simulink model "Senorless"  (R2023a)
settings: Solver=FixedStepDiscrete  StartTime=0.0  StopTime=2  FixedStep=1/FOC_FRQ  RelTol=1e-3
values from neighbouring files (symbols this model uses):
  ADC_REF = 3.6    [Senorless.sldd]
  ADC_SAMPLE_MAX = 32767.0    [Senorless.sldd]
  AMP_GAIN = 32.0    [Senorless.sldd]
  CURR_INPUT = 3276.0    [Senorless.sldd]
  CURR_KI = 380.0    [Senorless.sldd]
  CURR_KP = 0.04    [Senorless.sldd]
  CURR_LIMIT = 1.1    [Senorless.sldd]
  CURR_OVER = 34.0    [Senorless.sldd]
  CURR_POINT_GAIN = 7.0    [Senorless.sldd]
  CURR_STEP = 32760.0    [Senorless.sldd]
  CURR_UNDER = 0.03    [Senorless.sldd]
  CURR_WIDTH = 250.0    [Senorless.sldd]
  FOC_FRQ = 36000.0    [Senorless.sldd]
  GAMMA = 32767.0    [Senorless.sldd]
  HFI_ID = 2.125    [Senorless.sldd]
  IMAX = 34.0    [Senorless.sldd]
  LPF_FRQ = 300.0    [Senorless.sldd]
  MOTOR_DAMPER = 8.3E-7    [Senorless.sldd]
  MOTOR_FLUX = 0.0012713112    [Senorless.sldd]
  MOTOR_INERTIA = 1.02E-6    [Senorless.sldd]
  MOTOR_LS = 1.8E-5    [Senorless.sldd]
  MOTOR_PN = 7.0    [Senorless.sldd]
  MOTOR_RS = 0.065    [Senorless.sldd]
  NS_COMP_UD = 0.531    [Senorless.sldd]
  PLL_LIMIT = 0.95    [Senorless.sldd]
  PLL_WIDTH = 500.0    [Senorless.sldd]
  PWM_FRQ = 96000000.0    [Senorless.sldd]
  RS_HUNT = 0.002    [Senorless.sldd]
  SMOK_FRQ = 1200.0    [Senorless.sldd]
  SPD_LIMIT = 0.8    [Senorless.sldd]
  SPD_LPF_LEVEL = 15.0    [Senorless.sldd]
  SPD_MAX = 8100.0    [Senorless.sldd]
  SPD_MIN = -8100.0    [Senorless.sldd]
  SPD_REDUCE = 380.0    [Senorless.sldd]
  SPD_STEP = 3.0    [Senorless.sldd]
  SPD_WIDTH = 10.0    [Senorless.sldd]
  TS_POINT_GAIN = 10.0    [Senorless.sldd]
  UDC = 17.0    [Senorless.sldd]
  UDC_GAIN = 21.0    [Senorless.sldd]
  UDC_POINT_GAIN = 10.0    [Senorless.sldd]
undefined symbols (not defined in the file or in its folder): curr_q_ki, curr_q_kp, DiscIntNeverNeededParam, magnitude, PLL_LPF_LEVEL, Udc
libraries: simulink x20, slpidlib x5, mcbcontrolslib x4, mcbplantlib x1, autolibpmsminterior x1, autolibpmsmexterior x1, spspowerguiLib x1
(part 3 of 7)

== system Senorless/FOC_PointModel/标志位 ==
  NS_Flag : Inport  PortDimensions=1
  Obs_Theta : Inport  Port=2
  Action Port : ActionPort  InitializeStates=reset  ActionPortLabel=case [ 3 ]:
  Constant1 : Constant  Value=0  OutDataTypeStr=int32
  Constant4 : Constant  Value=0  OutDataTypeStr=int16
  Constant8 : Constant  Value=0  OutDataTypeStr=int16
  Data Store Write : DataStoreWrite  DataStoreName=NS_Flag  IndexOptions=Index vector (dialog)  Indices=1  OutputSizes=1
  Data Type Conversion1 : DataTypeConversion  Commented=on  OutDataTypeStr=int32  SaturateOnIntegerOverflow=off
  Data Type Conversion2 : DataTypeConversion  Commented=on  OutDataTypeStr=int32  SaturateOnIntegerOverflow=off
  Display : Display
  Shift Arithmetic : ArithShift  Commented=on  BitShiftNumber=-16
  Sign : Signum
  积分器 : Subsystem  Commented=on
      settings: MinAlgLoopOccurrences=on
  Theta : Outport
  Iq : Outport  Port=2
  Id : Outport  Port=3
  wires:
  Data Type Conversion1/1 -> 积分器/2(Xo)
  Data Type Conversion2/1 -> Shift Arithmetic/1
  Shift Arithmetic/1 -> 积分器/1(input)
  Constant8/1 -> Iq/1
  Constant4/1 -> Id/1
  Obs_Theta/1 -> Theta/1
  NS_Flag/1 -> Sign/1
  Sign/1 -> Display/1, Data Store Write/1

== system Senorless/FOC_PointModel/电压限转速 ==
  note: 通过实时检测母线电压，调整最大转速
  Udc_Ref : Inport
  SPD_Ref : Inport  Port=2
  Constant1 : Constant  Value=SPD_REDUCE  OutDataTypeStr=int32
  Constant2 : Constant  Value=2  OutDataTypeStr=int16
  Constant3 : Constant  Value=0  OutDataTypeStr=int16
  Constant6 : Constant  Value=SPD_MAX  OutDataTypeStr=int32
  Constant7 : Constant  Value=SPD_MIN  OutDataTypeStr=int32
  Data Store Read1 : DataStoreRead  DataStoreName=Uout_Max  IndexOptions=Index vector (dialog)  Indices=1  OutputSizes=1
  Data Store Read2 : DataStoreRead  DataStoreName=Uout_Max  IndexOptions=Index vector (dialog)  Indices=1  OutputSizes=1
  Data Store Read3 : DataStoreRead  DataStoreName=Uout_Max  IndexOptions=Index vector (dialog)  Indices=1  OutputSizes=1
  Product : Product  OutDataTypeStr=int32  RndMeth=Zero
  Product4 : Product  OutDataTypeStr=int32
  Saturation Dynamic1 : simulink/Discontinuities/Saturation Dynamic  OutMin=[]  OutMax=[]  OutDataTypeStr=Inherit: Same as second input  OutDataType=fixdt(1, 16)  OutScaling=2^-10  RndMeth=Zero  DoSatur=off
  Saturation Dynamic2 : simulink/Discontinuities/Saturation Dynamic  OutMin=[]  OutMax=[]  OutDataTypeStr=Inherit: Same as second input  OutDataType=fixdt(1, 16)  OutScaling=2^-10  RndMeth=Zero  DoSatur=off
  Shift Arithmetic : ArithShift  BitShiftNumber=15
  Sum : Sum  Inputs=-+  OutDataTypeStr=int16  RndMeth=Zero
  Sum1 : Sum  Inputs=-+  OutDataTypeStr=int16  RndMeth=Zero
  Sum2 : Sum  Inputs=+-  RndMeth=Zero
  out : Outport
  wires:
  Product4/1 -> Shift Arithmetic/1
  Sum/1 -> Saturation Dynamic1/2
  Shift Arithmetic/1 -> Sum/1
  SPD_Ref/1 -> Saturation Dynamic2/2
  Udc_Ref/1 -> Product4/2
  Sum2/1 -> Saturation Dynamic2/1
  Saturation Dynamic2/1 -> out/1
  Constant7/1 -> Saturation Dynamic2/3
  Constant1/1 -> Product/1
  Saturation Dynamic1/1 -> Product/2
  Constant6/1 -> Sum2/1
  Product/1 -> Sum2/2
  Data Store Read3/1 -> Product4/1
  Sum1/1 -> Sum/2
  Constant2/1 -> Sum1/1
  Data Store Read1/1 -> Sum1/2
  Constant3/1 -> Saturation Dynamic1/3
  Data Store Read2/1 -> Saturation Dynamic1/1

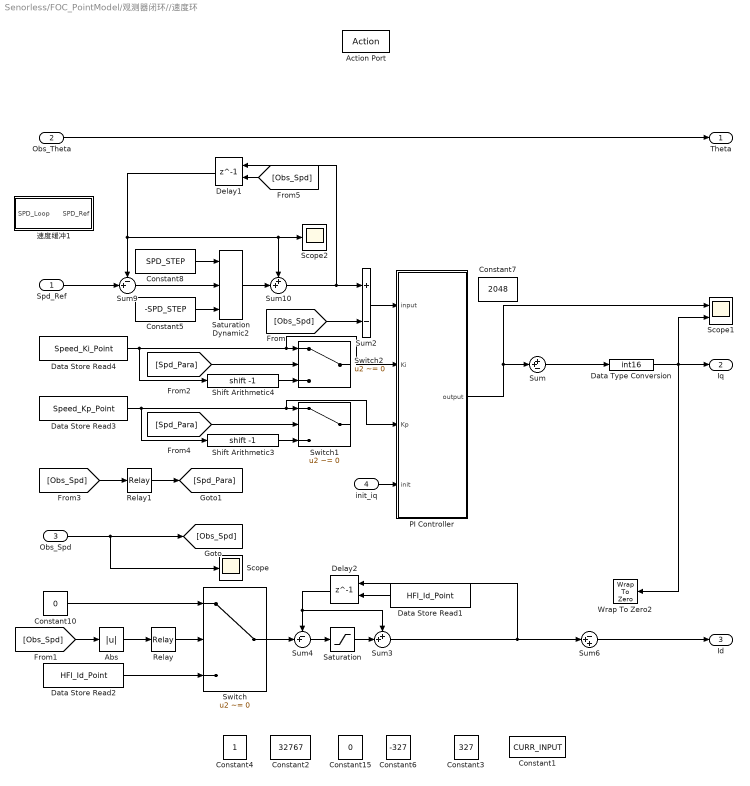
== system Senorless/FOC_PointModel/观测器闭环//速度环 ==
  Spd_Ref : Inport
  Obs_Theta : Inport  Port=2
  Obs_Spd : Inport  Port=3
  init_iq : Inport  Port=4
  Action Port : ActionPort  InitializeStates=reset  ActionPortLabel=case [ 4 ]:
  Abs : Abs  SaturateOnIntegerOverflow=off
  Constant1 : Constant  Value=CURR_INPUT  OutDataTypeStr=int16
  Constant10 : Constant  Value=0  OutDataTypeStr=int16
  Constant15 : Constant  Value=0  OutDataTypeStr=int16
  Constant2 : Constant  Value=32767  OutDataTypeStr=int16
  Constant3 : Constant  Value=327  OutDataTypeStr=int16
  Constant4 : Constant  OutDataTypeStr=int16
  Constant5 : Constant  Value=-SPD_STEP  OutDataTypeStr=int32
  Constant6 : Constant  Value=-327  OutDataTypeStr=int16
  Constant7 : Constant  Value=2048  OutDataTypeStr=int16
  Constant8 : Constant  Value=SPD_STEP  OutDataTypeStr=int32
  Data Store Read1 : DataStoreRead  DataStoreName=HFI_Id_Point  IndexOptions=Index vector (dialog)  Indices=1  OutputSizes=1
  Data Store Read2 : DataStoreRead  DataStoreName=HFI_Id_Point  IndexOptions=Index vector (dialog)  Indices=1  OutputSizes=1
  Data Store Read3 : DataStoreRead  DataStoreName=Speed_Kp_Point  IndexOptions=Index vector (dialog)  Indices=1  OutputSizes=1
  Data Store Read4 : DataStoreRead  DataStoreName=Speed_Ki_Point  IndexOptions=Index vector (dialog)  Indices=1  OutputSizes=1
  Data Type Conversion : DataTypeConversion  OutDataTypeStr=int16  SaturateOnIntegerOverflow=off
  Delay1 : Delay  DelayLength=1  InitialConditionSource=Input port
      settings: InputPortMap=u0,p4
  Delay2 : Delay  DelayLength=1  InitialConditionSource=Input port
      settings: InputPortMap=u0,p4
  PI Controller : Subsystem
      settings: MinAlgLoopOccurrences=on
  Relay : Relay  OnSwitchValue=1700  OffSwitchValue=1300  OnOutputValue=boolean(1)  OffOutputValue=boolean(0)  OutDataTypeStr=boolean
  Relay1 : Relay  OnSwitchValue=150  OffSwitchValue=100  OnOutputValue=boolean(1)  OffOutputValue=boolean(0)  OutDataTypeStr=boolean
  Saturation : Saturate  UpperLimit=16384  LowerLimit=-1
  Saturation Dynamic2 : simulink/Discontinuities/Saturation Dynamic  OutMin=[]  OutMax=[]  OutDataTypeStr=Inherit: Same as second input  OutDataType=fixdt(1, 16)  OutScaling=2^-10  RndMeth=Zero  DoSatur=off
  Scope : Scope
  Scope1 : Scope  NumInputPorts=2
  Scope2 : Scope
  Shift Arithmetic3 : ArithShift  BitShiftNumber=-1
  Shift Arithmetic4 : ArithShift  BitShiftNumber=-1
  Sum : Sum  Inputs=++-  RndMeth=Zero
  Sum10 : Sum  Inputs=++|  OutDataTypeStr=int32  RndMeth=Zero
  Sum2 : Sum  Inputs=+-  AccumDataTypeStr=int32  OutDataTypeStr=int16  RndMeth=Zero
  Sum3 : Sum  Inputs=++|  OutDataTypeStr=int16  RndMeth=Zero
  Sum4 : Sum  Inputs=-+|  OutDataTypeStr=int16  RndMeth=Zero
  Sum6 : Sum  Inputs=-++  OutDataTypeStr=int16  RndMeth=Zero
  Sum9 : Sum  Inputs=-+|  OutDataTypeStr=int32  RndMeth=Zero
  Switch : Switch  Criteria=u2 ~= 0  Threshold=1500  OutDataTypeStr=int16  RndMeth=Zero  SaturateOnIntegerOverflow=off  InputSameDT=off
  Switch1 : Switch  Criteria=u2 ~= 0  Threshold=100  SaturateOnIntegerOverflow=off  InputSameDT=off
  Switch2 : Switch  Criteria=u2 ~= 0  Threshold=100  SaturateOnIntegerOverflow=off  InputSameDT=off
  Wrap To Zero2 : simulink/Discontinuities/Wrap To Zero  Threshold=int16(0)
  速度缓冲1 : Stateflow chart  TreatAsAtomicUnit=on
  Theta : Outport  InitialOutput=uint16(0)
  Iq : Outport  Port=2  InitialOutput=int16(0)
  Id : Outport  Port=3  InitialOutput=int16(0)
  wires:
  Obs_Theta/1 -> Theta/1
  Sum2/1 -> PI Controller/1(input)
  Saturation Dynamic2/1 -> Sum10/2
  Delay1/1 -> Sum10/1, Scope2/1, Sum9/1
  Sum9/1 -> Saturation Dynamic2/2
  Constant8/1 -> Saturation Dynamic2/1
  Constant5/1 -> Saturation Dynamic2/3
  [Obs_Spd] -> Abs/1
  Relay/1 -> Switch/2
  Shift Arithmetic4/1 -> Switch2/3
  Shift Arithmetic3/1 -> Switch1/3
  Data Type Conversion/1 -> Wrap To Zero2/1, Scope1/2, Iq/1
  Sum/1 -> Data Type Conversion/1
  PI Controller/1(output) -> Scope1/1, Sum/2
  Sum3/1 -> Sum6/2, Delay2/1
  Sum4/1 -> Saturation/1
  Saturation/1 -> Sum3/2
  Delay2/1 -> Sum3/1, Sum4/1
  [Obs_Spd] -> Sum2/2
  Switch/1 -> Sum4/2
  [Obs_Spd] -> Relay1/1
  [Spd_Para] -> Switch2/2
  [Spd_Para] -> Switch1/2
  Relay1/1 -> [Spd_Para]
  Constant10/1 -> Switch/1
  Data Store Read4/1 -> Shift Arithmetic4/1, PI Controller/2(Ki), Switch2/1
  Data Store Read3/1 -> PI Controller/3(Kp), Switch1/1, Shift Arithmetic3/1
  Data Store Read2/1 -> Switch/3
  Data Store Read1/1 -> Delay2/2
  Spd_Ref/1 -> Sum9/2
  Sum10/1 -> Delay1/1, Sum2/1
  [Obs_Spd] -> Delay1/2
  init_iq/1 -> PI Controller/4(init)
  Obs_Spd/1 -> [Obs_Spd], Scope/1
  Sum6/1 -> Id/1
  Abs/1 -> Relay/1

== system Senorless/FOC_PointModel/识别初始位置 ==
  Obs_Theta : Inport
  Action Port : ActionPort  InitializeStates=reset  ActionPortLabel=case [ 1 ]:
  Constant1 : Constant  Value=0  OutDataTypeStr=int16
  Constant2 : Constant  Value=0  OutDataTypeStr=int16
  Theta : Outport
  Iq : Outport  Port=2
  Id : Outport  Port=3
  wires:
  Obs_Theta/1 -> Theta/1
  Constant1/1 -> Iq/1
  Constant2/1 -> Id/1

== system Senorless/FOC_PointModel/Err/PLL_LPF1 ==
  note: y(n)=ax(n)+(1−a)y(n−1)
  note: a =(ω c​ T s​ )/(1+ω c​ T s​ )
  input : Inport
  Constant1 : Constant  Value=15  OutDataTypeStr=int16
  Constant5 : Constant  OutDataTypeStr=int16
  Product10 : Product  OutDataTypeStr=int32
  Product11 : Product  OutDataTypeStr=int32  RndMeth=Zero
  Shift Arithmetic1 : ArithShift  BitShiftNumber=-4
  Shift Arithmetic9 : ArithShift  BitShiftNumber=4
  Sum10 : Sum  Inputs=-+
  Sum11 : Sum  OutDataTypeStr=int32  RndMeth=Zero
  Unit Delay9 : UnitDelay  SampleTime=-1  HasFrameUpgradeWarning=on
  output : Outport
  wires:
  input/1 -> Product10/2
  Unit Delay9/1 -> Product11/1
  Product10/1 -> Sum11/2
  Product11/1 -> Sum11/1
  Sum10/1 -> Product10/1
  Shift Arithmetic1/1 -> Sum10/2
  Shift Arithmetic9/1 -> Unit Delay9/1, output/1
  Sum11/1 -> Shift Arithmetic9/1
  Constant5/1 -> Shift Arithmetic1/1
  Constant1/1 -> Product11/2, Sum10/1

== system Senorless/FOC_PointModel/Err/闭环错误判断 ==
  Curr_Err : Inport
  Curr_Max : Inport  Port=2
  Obs_SPD : Inport  Port=3
  Udc_Ref : Inport  Port=4
  Enable : EnablePort  StatesWhenEnabling=reset
  Constant : Constant  Value=16384  OutDataTypeStr=int32
  Constant1 : Constant  Value=-100  OutDataTypeStr=int16
  Data Store Read : DataStoreRead  DataStoreName=FOC_FRQ_Point  IndexOptions=Index vector (dialog)  Indices=1  OutputSizes=1
  Data Store Read7 : DataStoreRead  DataStoreName=Curr_Under  IndexOptions=Index vector (dialog)  Indices=1  OutputSizes=1
  Data Type Conversion12 : DataTypeConversion  OutDataTypeStr=int32  SaturateOnIntegerOverflow=off
  Data Type Conversion13 : DataTypeConversion  OutDataTypeStr=uint8  SaturateOnIntegerOverflow=off
  If1 : If
  Logical Operator : Logic  Operator=OR  Inputs=3  AllPortsSameDT=off  OutDataTypeStr=boolean
  Merge3 : Merge
  OR1 : Logic  Operator=OR  AllPortsSameDT=off  OutDataTypeStr=boolean
  Relational Operator1 : RelationalOperator  Operator=<  OutDataTypeStr=boolean  RndMeth=Zero  InputSameDT=off
  Relational Operator2 : RelationalOperator  Operator=<  OutDataTypeStr=boolean  RndMeth=Zero  InputSameDT=off
  Relational Operator3 : RelationalOperator  OutDataTypeStr=boolean  RndMeth=Zero  InputSameDT=off
  Relational Operator4 : RelationalOperator  Operator=<  OutDataTypeStr=boolean  RndMeth=Zero  InputSameDT=off
  SUM : Subsystem
  Scope : Scope
  Scope1 : Scope
  Scope2 : Scope
  Unit Delay : UnitDelay  SampleTime=-1  HasFrameUpgradeWarning=on
  ZERO : Subsystem
  半秒的意思 : ArithShift  BitShiftNumber=1
  Run_Err : Outport
  wires:
  If1/2 -> ZERO/Action
  Data Store Read/1 -> 半秒的意思/1
  Data Store Read7/1 -> Relational Operator1/2
  Data Type Conversion12/1 -> SUM/1(in)
  Logical Operator/1 -> Data Type Conversion12/1, Data Type Conversion13/1
  ZERO/1(out) -> Merge3/2
  Relational Operator3/1 -> OR1/2, Scope2/1
  Curr_Max/1 -> Relational Operator1/1
  Curr_Err/1 -> OR1/1
  If1/1 -> SUM/Action
  Constant1/1 -> Relational Operator2/2
  Merge3/1 -> Scope1/1, Relational Operator3/1
  OR1/1 -> Scope/1, Run_Err/1
  Data Type Conversion13/1 -> If1/1
  SUM/1(out) -> Merge3/1
  半秒的意思/1 -> Relational Operator3/2
  Relational Operator1/1 -> Logical Operator/2
  Relational Operator4/1 -> Logical Operator/1
  Constant/1 -> Relational Operator4/2
  Udc_Ref/1 -> Relational Operator4/1
  Obs_SPD/1 -> Unit Delay/1
  Unit Delay/1 -> Relational Operator2/1

== system Senorless/FOC_PointModel/NS辨识/max ==
  input : Inport
  Enable : EnablePort  StatesWhenEnabling=reset
  Sum : Sum  Inputs=|++  OutDataTypeStr=int32  RndMeth=Zero
  Unit Delay : UnitDelay  SampleTime=-1  HasFrameUpgradeWarning=on
  output : Outport
  wires:
  Unit Delay/1 -> Sum/2
  Sum/1 -> output/1, Unit Delay/1
  input/1 -> Sum/1

== system Senorless/FOC_PointModel/NS辨识/min ==
  input : Inport
  Enable : EnablePort  StatesWhenEnabling=reset
  Sum : Sum  Inputs=|++  OutDataTypeStr=int32  RndMeth=Zero
  Unit Delay : UnitDelay  SampleTime=-1  HasFrameUpgradeWarning=on
  output : Outport
  wires:
  input/1 -> Sum/1
  Sum/1 -> Unit Delay/1, output/1
  Unit Delay/1 -> Sum/2

== system Senorless/FOC_PointModel/NS辨识/sincos_4096 ==
  theta : Inport
  Constant1 : Constant  Value=128  OutDataTypeStr=uint16
  Constant3 : Constant  Value=16384+128  OutDataTypeStr=uint16
  Shift Arithmetic : ArithShift  BitShiftNumber=4
  Shift Arithmetic1 : ArithShift  BitShiftNumber=4
  Sin : Lookup_n-D  NumberOfTableDimensions=1  BreakpointsSpecification=Even spacing  BreakpointsForDimension1=uint16(linspace(0,511,512))  BreakpointsForDimension1DataTypeStr=uint16  IndexSearchMethod=Linear search  BeginIndexSearchUsingPreviousIndexResult=on  UseOneInputPortForAllInputData=on  Table=int16(32767*sin(linspace(0,2*pi,4096)))  TableDataTypeStr=int16  IntermediateResultsDataTypeStr=int32  InterpMethod=Flat  ExtrapMethod=Clip  RemoveProtectionInput=on  ApplyFullPrecisionForLinearInterpolation=on  InternalRulePriority=Speed  OutDataTypeStr=int16  RndMeth=Zero  FractionDataTypeStr=fixdt(1,16,0)  InputSameDT=off
  Sin1 : Lookup_n-D  NumberOfTableDimensions=1  BreakpointsSpecification=Even spacing  BreakpointsForDimension1=uint16(linspace(0,511,512))  BreakpointsForDimension1DataTypeStr=uint16  IndexSearchMethod=Linear search  BeginIndexSearchUsingPreviousIndexResult=on  UseOneInputPortForAllInputData=on  Table=int16(32767*sin(linspace(0,2*pi,4096)))  TableDataTypeStr=int16  IntermediateResultsDataTypeStr=int32  InterpMethod=Flat  ExtrapMethod=Clip  RemoveProtectionInput=on  ApplyFullPrecisionForLinearInterpolation=on  InternalRulePriority=Speed  OutDataTypeStr=int16  RndMeth=Zero  FractionDataTypeStr=fixdt(1,16,0)  InputSameDT=off
  Sin2 : Lookup_n-D  Commented=on  NumberOfTableDimensions=1  BreakpointsSpecification=Even spacing  BreakpointsForDimension1=uint16(linspace(0,511,512))  BreakpointsForDimension1DataTypeStr=uint16  IndexSearchMethod=Linear search  BeginIndexSearchUsingPreviousIndexResult=on  UseOneInputPortForAllInputData=on  Table=|  TableDataTypeStr=int16  IntermediateResultsDataTypeStr=int32  InterpMethod=Flat  ExtrapMethod=Clip  RemoveProtectionInput=on  ApplyFullPrecisionForLinearInterpolation=on  InternalRulePriority=Speed  OutDataTypeStr=int16  RndMeth=Zero  FractionDataTypeStr=fixdt(1,16,0)  InputSameDT=off
      | int16([
      |  0 ,   402 ,   804 ,  1207 ,  1609 , ...
      |       2011 ,  2412 ,  2814 ,  3214 ,  3615 , ...
      |       4015 ,  4414 ,  4812 ,  5210 ,  5607 , ...
      |       6003 ,  6398 ,  6793 ,  7186 ,  7578 , ...
      |       7969 ,  8359 ,  8747 ,  9135 ,  9521 , ...
      |       9905 , 10288 , 10669 , 11049 , 11427 , ...
      |      11804 , 12178 , 12551 , 12922 , 13291 , ...
      |      13658 , 14022 , 14385 , 14746 , 15104 , ...
      |      15460 , 15814 , 16165 , 16514 , 16860 , ...
      |      17204 , 17546 , 17884 , 18220 , 18553 , ...
      |      18884 , 19211 , 19536 , 19857 , 20176 , ...
      |      20492 , 20804 , 21114 , 21420 , 21723 , ...
      |      22023 , 22319 , 22612 , 22902 , 23188 , ...
      |      23470 , 23750 , 24025 , 24297 , 24565 , ...
      |      24830 , 25090 , 25347 , 25601 , 25850 , ...
      |      26095 , 26337 , 26574 , 26808 , 27037 , ...
      |      27263 , 27484 , 27701 , 27914 , 28123 , ...
      |      28327 , 28527 , 28723 , 28915 , 29102 , ...
      |      29285 , 29463 , 29637 , 29806 , 29971 , ...
      |      30132 , 30288 , 30439 , 30586 , 30728 , ...
      |      30865 , 30998 , 31126 , 31250 , 31368 , ...
      |      31482 , 31592 , 31696 , 31796 , 31891 , ...
      |      31981 , 32066 , 32146 , 32222 , 32293 , ...
      |      32359 , 32419 , 32476 , 32527 , 32573 , ...
      |      32614 , 32651 , 32682 , 32709 , 32730 , ...
      |      32747 , 32759 , 32766 , 32767 , 32764 , ...
      |      32756 , 32743 , 32725 , 32703 , 32675 , ...
      |      32642 , 32604 , 32562 , 32514 , 32462 , ...
      |      32405 , 32343 , 32275 , 32204 , 32127 , ...
      |      32045 , 31959 , 31867 , 31771 , 31670 , ...
      |      31565 , 31454 , 31339 , 31219 , 31095 , ...
      |      30965 , 30831 , 30693 , 30549 , 30402 , ...
      |      30249 , 30092 , 29930 , 29764 , 29594 , ...
      |      29419 , 29239 , 29055 , 28867 , 28674 , ...
      |      28478 , 28276 , 28071 , 27861 , 27647 , ...
      |      27429 , 27207 , 26980 , 26750 , 26515 , ...
      |      26277 , 26034 , 25788 , 25538 , 25284 , ...
      |      25026 , 24764 , 24498 , 24229 , 23956 , ...
      |      23680 , 23400 , 23117 , 22830 , 22539 , ...
      |      22245 , 21948 , 21647 , 21344 , 21037 , ...
      |      20726 , 20413 , 20097 , 19777 , 19455 , ...
      |      19130 , 18801 , 18470 , 18136 , 17800 , ...
      |      17461 , 17119 , 16774 , 16427 , 16078 , ...
      |      15726 , 15371 , 15015 , 14656 , 14295 , ...
      |      13931 , 13566 , 13199 , 12829 , 12458 , ...
      |      12085 , 11710 , 11333 , 10954 , 10574 , ...
      |      10192 ,  9809 ,  9424 ,  9038 ,  8650 , ...
      |       8262 ,  7871 ,  7480 ,  7088 ,  6694 , ...
      |       6300 ,  5904 ,  5508 ,  5111 ,  4713 , ...
      |       4314 ,  3915 ,  3515 ,  3114 ,  2713 , ...
      |       2312 ,  1910 ,  1508 ,  1106 ,   704 , ...
      |        301 ,  -100 ,  -503 ,  -905 , -1307 , ...
      |      -1709 , -2111 , -2513 , -2914 , -3315 , ...
      |      -3715 , -4114 , -4513 , -4912 , -5309 , ...
      |      -5706 , -6102 , -6497 , -6891 , -7284 , ...
      |      -7676 , -8067 , -8456 , -8844 , -9231 , ...
      |      -9617 ,-10001 ,-10383 ,-10764 ,-11144 , ...
      |     -11521 ,-11897 ,-12271 ,-12644 ,-13014 , ...
      |     -13383 ,-13749 ,-14113 ,-14475 ,-14835 , ...
      |     -15193 ,-15549 ,-15902 ,-16253 ,-16601 , ...
      |     -16947 ,-17290 ,-17630 ,-17968 ,-18304 , ...
      |     -18636 ,-18966 ,-19293 ,-19616 ,-19937 , ...
      |     -20255 ,-20570 ,-20882 ,-21191 ,-21496 , ...
      |     -21798 ,-22097 ,-22393 ,-22685 ,-22973 , ...
      |     -23259 ,-23541 ,-23819 ,-24093 ,-24364 , ...
      |     -24632 ,-24895 ,-25155 ,-25411 ,-25663 , ...
      |     -25912 ,-26156 ,-26397 ,-26633 ,-26866 , ...
      |     -27094 ,-27318 ,-27538 ,-27755 ,-27966 , ...
      |     -28174 ,-28377 ,-28577 ,-28771 ,-28962 , ...
      |     -29148 ,-29330 ,-29507 ,-29680 ,-29848 , ...
      |     -30012 ,-30171 ,-30326 ,-30476 ,-30622 , ...
      |     -30763 ,-30899 ,-31031 ,-31157 ,-31280 , ...
      |     -31397 ,-31510 ,-31618 ,-31721 ,-31820 , ...
      |     -31914 ,-32003 ,-32087 ,-32166 ,-32240 , ...
      |     -32310 ,-32374 ,-32434 ,-32489 ,-32539 , ...
      |     -32584 ,-32624 ,-32659 ,-32689 ,-32715 , ...
      |     -32735 ,-32750 ,-32761 ,-32767 ,-32767 , ...
      |     -32763 ,-32754 ,-32739 ,-32720 ,-32696 , ...
      |     -32667 ,-32633 ,-32594 ,-32550 ,-32502 , ...
      |     -32448 ,-32390 ,-32326 ,-32258 ,-32185 , ...
      |     -32107 ,-32024 ,-31936 ,-31844 ,-31747 , ...
      |     -31644 ,-31538 ,-31426 ,-31310 ,-31189 , ...
      |     -31063 ,-30932 ,-30797 ,-30657 ,-30513 , ...
      |     -30364 ,-30210 ,-30052 ,-29889 ,-29722 , ...
      |     -29550 ,-29374 ,-29194 ,-29009 ,-28819 , ...
      |     -28626 ,-28428 ,-28225 ,-28019 ,-27808 , ...
      |     -27593 ,-27374 ,-27150 ,-26923 ,-26692 , ...
      |     -26456 ,-26217 ,-25973 ,-25726 ,-25475 , ...
      |     -25219 ,-24961 ,-24698 ,-24432 ,-24161 , ...
      |     -23888 ,-23610 ,-23330 ,-23045 ,-22757 , ...
      |     -22466 ,-22171 ,-21873 ,-21572 ,-21267 , ...
      |     -20959 ,-20648 ,-20334 ,-20017 ,-19697 , ...
      |     -19374 ,-19048 ,-18719 ,-18387 ,-18052 , ...
      |     -17715 ,-17375 ,-17033 ,-16688 ,-16340 , ...
      |     -15990 ,-15637 ,-15282 ,-14925 ,-14566 , ...
      |     -14204 ,-13840 ,-13474 ,-13106 ,-12737 , ...
      |     -12365 ,-11991 ,-11616 ,-11238 ,-10859 , ...
      |     -10479 ,-10097 , -9713 , -9328 , -8941 , ...
      |      -8553 , -8164 , -7774 , -7382 , -6989 , ...
      |      -6596 , -6201 , -5805 , -5409 , -5011 , ...
      |      -4613 , -4214 , -3815 , -3415 , -3014 , ...
      |      -2613 , -2212 , -1810 , -1408 , -1006 , ...
      |       -603 ,  -201 ...
      |     ])
  Sin3 : Lookup_n-D  Commented=on  NumberOfTableDimensions=1  BreakpointsSpecification=Even spacing  BreakpointsForDimension1=uint16(linspace(0,511,512))  BreakpointsForDimension1DataTypeStr=uint16  IndexSearchMethod=Linear search  BeginIndexSearchUsingPreviousIndexResult=on  UseOneInputPortForAllInputData=on  Table=int16(32767*sin(linspace(0,2*pi,512)))  TableDataTypeStr=int16  IntermediateResultsDataTypeStr=int32  InterpMethod=Flat  ExtrapMethod=Clip  RemoveProtectionInput=on  ApplyFullPrecisionForLinearInterpolation=on  InternalRulePriority=Speed  OutDataTypeStr=int16  RndMeth=Zero  FractionDataTypeStr=fixdt(1,16,0)  InputSameDT=off
  Sum1 : Sum  Inputs=|++
  Sum2 : Sum  Inputs=|++
  theta1 : InportShadow
  cos : Outport
  sin : Outport  Port=2
  wires:
  Shift Arithmetic/1 -> Sin1/1
  Sum2/1 -> Shift Arithmetic/1
  Constant3/1 -> Sum2/2
  Shift Arithmetic1/1 -> Sin/1
  theta1/1 -> Sum2/1
  theta/1 -> Sum1/1
  Sin/1 -> sin/1
  Sin1/1 -> cos/1
  Sum1/1 -> Shift Arithmetic1/1
  Constant1/1 -> Sum1/2

== system Senorless/FOC_PointModel/NS辨识/加速积分角度 ==
  Acc : Inport
  Data Type Conversion : DataTypeConversion  Commented=on  OutDataTypeStr=int16  SaturateOnIntegerOverflow=off
  Data Type Conversion1 : DataTypeConversion  Commented=on  OutDataTypeStr=int16  SaturateOnIntegerOverflow=off
  Data Type Conversion2 : DataTypeConversion  OutDataTypeStr=uint16  SaturateOnIntegerOverflow=off
  Data Type Conversion3 : DataTypeConversion  OutDataTypeStr=int32  SaturateOnIntegerOverflow=off
  Freq1 : InportShadow
  Gain6 : Gain  Commented=on  Gain=65535  OutDataTypeStr=int32  RndMeth=Zero
  Scope1 : Scope  Commented=on
  Scope2 : Scope  Commented=on
  Shift Arithmetic : ArithShift  BitShiftNumber=-16
  初始值1 : Constant  Commented=on  Value=0  OutDataTypeStr=int32
  初始值3 : Constant  Commented=on  Value=0  OutDataTypeStr=int32
  积分器 : Subsystem  Commented=on
  积分器2 : Subsystem  Commented=on
  积分器3 : Subsystem
      settings: MinAlgLoopOccurrences=on
  积分器4 : Subsystem
      settings: MinAlgLoopOccurrences=on
  积分增益 : Constant  Commented=on  Value=32767  OutDataTypeStr=int32
  积分增益1 : Constant  Commented=on  Value=32767  OutDataTypeStr=int32
  这是积分增益缩小 : ArithShift  Commented=on  BitShiftNumber=15
  这是积分增益缩小1 : ArithShift  Commented=on  BitShiftNumber=15
  Theta : Outport
  wires:
  Data Type Conversion1/1 -> Gain6/1
  Gain6/1 -> 积分器/2(input)
  积分增益/1 -> 积分器/1(K_p)
  初始值1/1 -> 积分器2/3(Xo)
  积分增益1/1 -> 积分器2/1(K_p)
  这是积分增益缩小1/1 -> Data Type Conversion/1
  积分器2/1(output) -> Scope1/1, 这是积分增益缩小/1
  积分器/1(output) -> Scope2/1, 积分器2/2(input)
  这是积分增益缩小/1 -> 这是积分增益缩小1/1
  Shift Arithmetic/1 -> 积分器3/1(input)
  Acc/1 -> Data Type Conversion3/1
  Freq1/1 -> Data Type Conversion1/1
  初始值3/1 -> 积分器/3(Xo)
  Data Type Conversion2/1 -> Theta/1
  积分器3/1(output) -> 积分器4/1(input)
  积分器4/1(output) -> Data Type Conversion2/1
  Data Type Conversion3/1 -> Shift Arithmetic/1

== system Senorless/FOC_PointModel/Observers/HFI ==
  HF : Inport
  ialpha : Inport  Port=2
  ibeta : Inport  Port=3
  Delay : Delay  DelayLength=1
  Delay1 : Delay  DelayLength=1
  HF1 : InportShadow
  Product4 : Product  OutDataTypeStr=int32  RndMeth=Zero
  Product5 : Product  OutDataTypeStr=int32  RndMeth=Zero
  Scope1 : Scope  NumInputPorts=3
  Scope10 : Scope  NumInputPorts=2
  Scope14 : Scope  NumInputPorts=3
  Shift Arithmetic4 : ArithShift  BitShiftNumber=1
  Shift Arithmetic5 : ArithShift  BitShiftNumber=1
  Sum2 : Sum  Inputs=|+-
  Sum3 : Sum  Inputs=|+-
  sin : Outport
  cos : Outport  Port=2
  wires:
  Sum2/1 -> Shift Arithmetic4/1
  ibeta/1 -> Sum2/1, Delay/1
  ialpha/1 -> Sum3/1, Delay1/1
  Product5/1 -> sin/1, Scope14/3, Scope10/2
  Product4/1 -> cos/1, Scope1/3, Scope10/1
  Sum3/1 -> Shift Arithmetic5/1
  Shift Arithmetic5/1 -> Scope1/2, Product4/2
  Delay1/1 -> Sum3/2
  Delay/1 -> Sum2/2
  Shift Arithmetic4/1 -> Product5/2, Scope14/2
  HF/1 -> Scope1/1, Product4/1
  HF1/1 -> Product5/1, Scope14/1

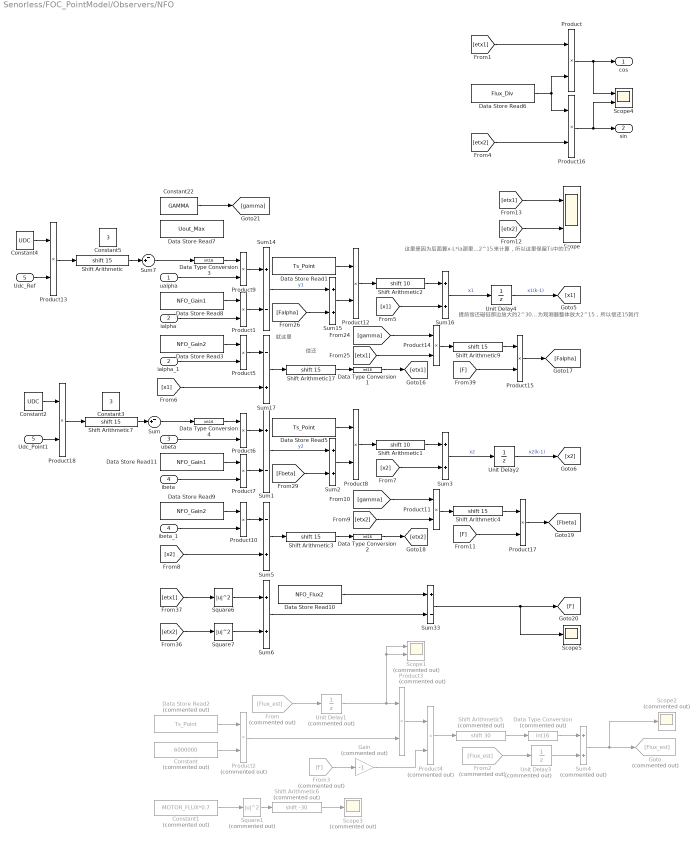
== system Senorless/FOC_PointModel/Observers/NFO ==
  note: 提前偿还磁链那边放大的2^30，因为观测器整体放大2^15，所以偿还15就行
  note: 偿还
  note: 就这里
  note: 这里是因为后面算x-L*ia那里需要再放大2^15来计算，所以这里保留Ts中的15
  ualpha : Inport
  ialpha : Inport  Port=2
  ubeta : Inport  Port=3
  ibeta : Inport  Port=4
  Udc_Ref : Inport  Port=5
  Constant : Constant  Commented=on  Value=6000000  OutDataTypeStr=int32
  Constant1 : Constant  Commented=on  Value=MOTOR_FLUX*0.7  OutDataTypeStr=single
  Constant2 : Constant  Value=UDC  OutDataTypeStr=int16
  Constant22 : Constant  Value=GAMMA  OutDataTypeStr=uint32
  Constant3 : Constant  Value=3  OutDataTypeStr=int16
  Constant4 : Constant  Value=UDC  OutDataTypeStr=int16
  Constant5 : Constant  Value=3  OutDataTypeStr=int16
  Data Store Read1 : DataStoreRead  DataStoreName=Ts_Point  IndexOptions=Index vector (dialog)  Indices=1  OutputSizes=1
  Data Store Read10 : DataStoreRead  DataStoreName=NFO_Flux2  IndexOptions=Index vector (dialog)  Indices=1  OutputSizes=1
  Data Store Read11 : DataStoreRead  DataStoreName=NFO_Gain1  IndexOptions=Index vector (dialog)  Indices=1  OutputSizes=1
  Data Store Read2 : DataStoreRead  Commented=on  DataStoreName=Ts_Point  IndexOptions=Index vector (dialog)  Indices=1  OutputSizes=1
  Data Store Read3 : DataStoreRead  DataStoreName=NFO_Gain2  IndexOptions=Index vector (dialog)  Indices=1  OutputSizes=1
  Data Store Read5 : DataStoreRead  DataStoreName=Ts_Point  IndexOptions=Index vector (dialog)  Indices=1  OutputSizes=1
  Data Store Read6 : DataStoreRead  DataStoreName=Flux_Div  IndexOptions=Index vector (dialog)  Indices=1  OutputSizes=1
  Data Store Read7 : DataStoreRead  DataStoreName=Uout_Max  IndexOptions=Index vector (dialog)  Indices=1  OutputSizes=1
  Data Store Read8 : DataStoreRead  DataStoreName=NFO_Gain1  IndexOptions=Index vector (dialog)  Indices=1  OutputSizes=1
  Data Store Read9 : DataStoreRead  DataStoreName=NFO_Gain2  IndexOptions=Index vector (dialog)  Indices=1  OutputSizes=1
  Data Type Conversion : DataTypeConversion  Commented=on  OutDataTypeStr=int16  SaturateOnIntegerOverflow=off
  Data Type Conversion{1..4} (4 alike) : DataTypeConversion  OutDataTypeStr=int16  SaturateOnIntegerOverflow=off
  From : From  Commented=on  GotoTag=Flux_est
  From2 : From  Commented=on  GotoTag=Flux_est
  From3 : From  Commented=on  GotoTag=F
  Gain : Gain  Commented=on  Gain=-1  OutDataTypeStr=int16  RndMeth=Zero
  Goto : Goto  Commented=on  GotoTag=Flux_est
  Product : Product
  Product{1,5..12,14..15,17} (12 alike) : Product  OutDataTypeStr=int32  RndMeth=Zero
  Product13 : Product  OutDataTypeStr=int32
  Product16 : Product
  Product18 : Product  OutDataTypeStr=int32
  Product2 : Product  Commented=on  OutDataTypeStr=int32  RndMeth=Zero
  Product3 : Product  Commented=on  OutDataTypeStr=int32  RndMeth=Zero
  Product4 : Product  Commented=on  OutDataTypeStr=int32  RndMeth=Zero
  Scope : Scope  NumInputPorts=2
  Scope1 : Scope  Commented=on  NumInputPorts=2
  Scope2 : Scope  Commented=on
  Scope3 : Scope  Commented=on
  Scope4 : Scope  NumInputPorts=2
  Scope5 : Scope
  Shift Arithmetic{,3..4,7,9,17} (6 alike) : ArithShift  BitShiftNumber=15
  Shift Arithmetic1 : ArithShift  BitShiftNumber=10
  Shift Arithmetic2 : ArithShift  BitShiftNumber=10
  Shift Arithmetic5 : ArithShift  Commented=on  BitShiftNumber=30
  Shift Arithmetic6 : ArithShift  Commented=on  BitShiftNumber=-30
  Square1 : Math  Commented=on  Operator=magnitude^2
  Square6 : Math  Operator=magnitude^2
  Square7 : Math  Operator=magnitude^2
  Sum : Sum  Inputs=-+|
  Sum1 : Sum  Inputs=+-  OutDataTypeStr=int32  RndMeth=Zero
  Sum14 : Sum  Inputs=+-  OutDataTypeStr=int32  RndMeth=Zero
  Sum{2..3,6,15..16} (5 alike) : Sum  OutDataTypeStr=int32  RndMeth=Zero
  Sum17 : Sum  Inputs=-+  OutDataTypeStr=int32  RndMeth=Zero
  Sum33 : Sum  Inputs=+-  OutDataTypeStr=int16  RndMeth=Zero
  Sum4 : Sum  Commented=on  OutDataTypeStr=int16  RndMeth=Zero
  Sum5 : Sum  Inputs=-+  OutDataTypeStr=int32  RndMeth=Zero
  Sum7 : Sum  Inputs=-+|
  Udc_Point1 : InportShadow  Port=5
  Unit Delay1 : UnitDelay  Commented=on  SampleTime=-1  HasFrameUpgradeWarning=on
  Unit Delay2 : UnitDelay  SampleTime=-1  HasFrameUpgradeWarning=on
  Unit Delay3 : UnitDelay  Commented=on  InitialCondition=4842  SampleTime=-1  HasFrameUpgradeWarning=on
  Unit Delay4 : UnitDelay  SampleTime=-1  HasFrameUpgradeWarning=on
  ialpha_1 : InportShadow  Port=2
  ibeta_1 : InportShadow  Port=4
  cos : Outport
  sin : Outport  Port=2
  wires:
  Sum3/1 -> Unit Delay2/1  "x2"
  [gamma] -> Product14/1
  Product17/1 -> [Fbeta]
  Unit Delay2/1 -> [x2]  "x2(k-1)"
  Data Store Read1/1 -> Product12/1
  [etx1] -> Scope/1
  [x1] -> Sum16/2
  Data Store Read9/1 -> Product10/1
  ialpha_1/1 -> Product5/2
  Product1/1 -> Sum14/2
  [x2] -> Sum5/2
  Constant22/1 -> [gamma]
  Shift Arithmetic4/1 -> Product17/1
  ubeta/1 -> Product6/2
  Sum6/1 -> Sum33/2
  Sum15/1 -> Product12/2
  Product12/1 -> Shift Arithmetic2/1
  Sum2/1 -> Product8/2
  Product8/1 -> Shift Arithmetic1/1
  [gamma] -> Product11/1
  [x2] -> Sum3/2
  ibeta/1 -> Product7/2
  Square6/1 -> Sum6/1
  Product7/1 -> Sum1/2
  Sum17/1 -> Shift Arithmetic17/1
  Data Store Read5/1 -> Product8/1
  ialpha/1 -> Product1/2
  [etx2] -> Scope/2
  Sum5/1 -> Shift Arithmetic3/1
  ualpha/1 -> Product9/2
  [F] -> Product17/2
  [Falpha] -> Sum15/2
  Product10/1 -> Sum5/1
  Product11/1 -> Shift Arithmetic4/1
  Sum16/1 -> Unit Delay4/1  "x1"
  Product5/1 -> Sum17/1
  Data Store Read8/1 -> Product1/1
  [etx2] -> Square7/1
  [etx2] -> Product11/2
  [Fbeta] -> Sum2/2
  Shift Arithmetic2/1 -> Sum16/1
  Unit Delay4/1 -> [x1]  "x1(k-1)"
  Product15/1 -> [Falpha]
  [etx1] -> Product14/2
  [etx1] -> Square6/1
  Shift Arithmetic3/1 -> Data Type Conversion2/1
  Shift Arithmetic1/1 -> Sum3/1
  [x1] -> Sum17/2
  ibeta_1/1 -> Product10/2
  Data Store Read11/1 -> Product7/1
  Sum14/1 -> Sum15/1  "y1"
  Shift Arithmetic17/1 -> Data Type Conversion1/1
  Sum1/1 -> Sum2/1  "y2"
  Data Store Read3/1 -> Product5/1
  Square7/1 -> Sum6/2
  Constant/1 -> Product2/2
  Data Store Read2/1 -> Product2/1
  Sum33/1 -> Scope5/1, [F]
  From3/1 -> Gain/1
  Product4/1 -> Shift Arithmetic5/1
  Unit Delay1/1 -> Scope1/2, Scope1/1, Product3/1
  From/1 -> Unit Delay1/1
  Product3/1 -> Product4/1
  Shift Arithmetic5/1 -> Data Type Conversion/1
  Gain/1 -> Product4/2
  Data Type Conversion/1 -> Sum4/1
  Unit Delay3/1 -> Sum4/2
  Sum4/1 -> Goto/1, Scope2/1
  From2/1 -> Unit Delay3/1
  Product2/1 -> Product3/2
  Constant1/1 -> Square1/1
  Square1/1 -> Shift Arithmetic6/1
  Shift Arithmetic6/1 -> Scope3/1
  Data Store Read10/1 -> Sum33/1
  Data Store Read6/1 -> Product16/1, Product/2
  Product/1 -> cos/1, Scope4/1
  Product16/1 -> sin/1, Scope4/2
  Product14/1 -> Shift Arithmetic9/1
  Data Type Conversion1/1 -> [etx1]
  Shift Arithmetic9/1 -> Product15/1
  [F] -> Product15/2
  Data Type Conversion2/1 -> [etx2]
  [etx1] -> Product/1
  [etx2] -> Product16/2
  Product13/1 -> Shift Arithmetic/1
  Constant4/1 -> Product13/1
  Udc_Ref/1 -> Product13/2
  Constant2/1 -> Product18/1
  Product18/1 -> Shift Arithmetic7/1
  Udc_Point1/1 -> Product18/2
  Product9/1 -> Sum14/1
  Product6/1 -> Sum1/1
  Data Type Conversion3/1 -> Product9/1
  Shift Arithmetic7/1 -> Sum/2
  Data Type Conversion4/1 -> Product6/1
  Sum/1 -> Data Type Conversion4/1
  Shift Arithmetic/1 -> Sum7/2
  Sum7/1 -> Data Type Conversion3/1

== system Senorless/FOC_PointModel/Observers/PLL ==
  note: 因为理论上Spd不会大于滤波器频率，除法范围在0-1，所以放大256倍
  sin : Inport
  cos : Inport  Port=2
  Bias : Bias  Bias=int32(1)  SaturateOnIntegerOverflow=off
  Constant : Constant  Value=32767  OutDataTypeStr=uint16
  Constant1 : Constant  Value=0  OutDataTypeStr=uint16
  Data Store Read1 : DataStoreRead  DataStoreName=NS_Flag  IndexOptions=Index vector (dialog)  Indices=1  OutputSizes=1
  Data Store Read6 : DataStoreRead  DataStoreName=DIV_LPF_FRQ  IndexOptions=Index vector (dialog)  Indices=1  OutputSizes=1
  Data Store Read7 : DataStoreRead  DataStoreName=PLL_Kp  IndexOptions=Index vector (dialog)  Indices=1  OutputSizes=1
  Data Store Read8 : DataStoreRead  DataStoreName=PLL_Ki  IndexOptions=Index vector (dialog)  Indices=1  OutputSizes=1
  Data Type Conversion8 : DataTypeConversion  OutDataTypeStr=uint16  SaturateOnIntegerOverflow=off
  PI Controller : Subsystem
      settings: MinAlgLoopOccurrences=on
  Product2 : Product  OutDataTypeStr=int32  RndMeth=Zero
  Product3 : Product  OutDataTypeStr=int32  RndMeth=Zero
  Product4 : Product  OutDataTypeStr=int32  RndMeth=Zero
  Scope : Scope
  Scope1 : Scope
  Scope3 : Scope
  Shift Arithmetic1 : ArithShift
  Shift Arithmetic10 : ArithShift  BitShiftNumber=-8
  Shift Arithmetic13 : ArithShift  BitShiftNumber=16
  Shift Arithmetic15 : ArithShift  BitShiftNumber=15
  Shift Arithmetic3 : ArithShift  BitShiftNumber=1
  Shift Arithmetic7 : ArithShift  BitShiftNumber=15
  Shift Arithmetic8 : ArithShift  BitShiftNumber=15
  Sin2_1 : MATLAB Function  Commented=on  TreatAsAtomicUnit=on
  Sum1 : Sum  Inputs=|+-  AccumDataTypeStr=uint16  OutDataTypeStr=uint16  RndMeth=Zero
  Sum3 : Sum  Inputs=-++  AccumDataTypeStr=uint16  OutDataTypeStr=uint16  RndMeth=Zero
  Sum4 : Sum  Inputs=+-
  Switch : Switch  SaturateOnIntegerOverflow=off  InputSameDT=off
  Unit Delay : UnitDelay  SampleTime=-1  HasFrameUpgradeWarning=on
  Unit Delay2 : UnitDelay  SampleTime=-1  HasFrameUpgradeWarning=on
  atan1 : Lookup_n-D  Commented=on  NumberOfTableDimensions=1  BreakpointsSpecification=Even spacing  BreakpointsForDimension1=[-5:5]  UseOneInputPortForAllInputData=on  Table=|  TableDataTypeStr=uint16  InterpMethod=Flat  RemoveProtectionInput=on  InternalRulePriority=Speed  OutDataTypeStr=uint16  RndMeth=Zero
      | uint16([...
      |         0, 64, 128, 192, 256, 320, 384, 448, 512, 576, 640, 704, 768, 832, 896, 960, ...
      |         1024, 1088, 1152, 1216, 1280, 1344, 1408, 1472, 1536, 1600, 1664, 1728, 1792, 1856, 1920, 1984, ...
      |         2048, 2112, 2176, 2240, 2304, 2368, 2432, 2496, 2560, 2624, 2688, 2752, 2816, 2880, 2944, 3008, ...
      |         3072, 3136, 3200, 3264, 3328, 3392, 3456, 3520, 3584, 3648, 3712, 3776, 3840, 3904, 3968, 4032, ...
      |         4096, 4160, 4224, 4288, 4352, 4416, 4480, 4544, 4608, 4672, 4736, 4800, 4864, 4928, 4992, 5056, ...
      |         5120, 5184, 5248, 5312, 5376, 5440, 5504, 5568, 5632, 5696, 5760, 5824, 5888, 5952, 6016, 6080, ...
      |         6144, 6208, 6272, 6336, 6400, 6464, 6528, 6592, 6656, 6720, 6784, 6848, 6912, 6976, 7040, 7104, ...
      |         7168, 7232, 7296, 7360, 7424, 7488, 7552, 7616, 7680, 7744, 7808, 7872, 7936, 8000, 8064, 8128, ...
      |         8192, 8256, 8320, 8384, 8448, 8512, 8576, 8640, 8704, 8768, 8832, 8896, 8960, 9024, 9088, 9152, ...
      |         9216, 9280, 9344, 9408, 9472, 9536, 9600, 9664, 9728, 9792, 9856, 9920, 9984, 10048, 10112, 10176, ...
      |         10240, 10304, 10368, 10432, 10496, 10560, 10624, 10688, 10752, 10816, 10880, 10944, 11008, 11072, 11136, 11200, ...
      |         11264, 11328, 11392, 11456, 11520, 11584, 11648, 11712, 11776, 11840, 11904, 11968, 12032, 12096, 12160, 12224, ...
      |         12288, 12352, 12416, 12480, 12544, 12608, 12672, 12736, 12800, 12864, 12928, 12992, 13056, 13120, 13184, 13248, ...
      |         13312, 13376, 13440, 13504, 13568, 13632, 13696, 13760, 13824, 13888, 13952, 14016, 14080, 14144, 14208, 14272, ...
      |         14336, 14400, 14464, 14528, 14592, 14656, 14720, 14784, 14848, 14912, 14976, 15040, 15104, 15168, 15232, 15296, ...
      |         15360, 15424, 15488, 15552, 15616, 15680, 15744, 15808, 15872, 15936, 16000, 16064, 16128, 16192, 16256, 16320])
  atan256 : Lookup_n-D  NumberOfTableDimensions=1  BreakpointsSpecification=Even spacing  BreakpointsForDimension1=[-5:5]  UseOneInputPortForAllInputData=on  Table=uint16(16384*atan(linspace(0,1,256)))  TableDataTypeStr=uint16  InterpMethod=Flat  RemoveProtectionInput=on  InternalRulePriority=Speed  OutDataTypeStr=uint16  RndMeth=Zero
  atan_1 : MATLAB Function  Commented=on  TreatAsAtomicUnit=on
  sincos_4096 : Subsystem
  积分器 : Subsystem
      settings: MinAlgLoopOccurrences=on
  Obs_Spd : Outport
  Obs_Theta : Outport  Port=2
  wires:
  积分器/1(output) -> Data Type Conversion8/1
  PI Controller/1(output) -> 积分器/1(input), Shift Arithmetic13/1  "Spd"
  [Theta_OS] -> Shift Arithmetic3/1
  [Theta_OS] -> Shift Arithmetic1/1
  Shift Arithmetic7/1 -> Sum4/1
  Product4/1 -> Shift Arithmetic7/1
  sin/1 -> Product4/1
  cos/1 -> Product3/2
  Shift Arithmetic8/1 -> Sum4/2
  Product3/1 -> Shift Arithmetic8/1
  Sum4/1 -> PI Controller/1(input)
  Product2/1 -> Shift Arithmetic15/1
  Data Store Read6/1 -> Shift Arithmetic10/1
  [Obs_Spd] -> Product2/2
  atan256/1 -> Scope3/1, [Theta_OS]
  Shift Arithmetic15/1 -> Bias/1
  Shift Arithmetic10/1 -> Product2/1
  Bias/1 -> atan256/1
  sincos_4096/1(cos) -> Product4/2
  sincos_4096/2(sin) -> Product3/1
  Sum3/1 -> Sum1/1
  Unit Delay/1 -> sincos_4096/1(theta)
  Unit Delay2/1 -> [Obs_Spd]
  Data Store Read7/1 -> PI Controller/2(Kp)
  Data Store Read8/1 -> PI Controller/3(Ki)
  Shift Arithmetic13/1 -> Obs_Spd/1, Scope/1, Unit Delay2/1
  Data Type Conversion8/1 -> Sum3/3
  Constant1/1 -> Switch/1
  Constant/1 -> Switch/3
  Data Store Read1/1 -> Switch/2
  Sum1/1 -> Scope1/1, Unit Delay/1, Obs_Theta/1
  Switch/1 -> Sum1/2

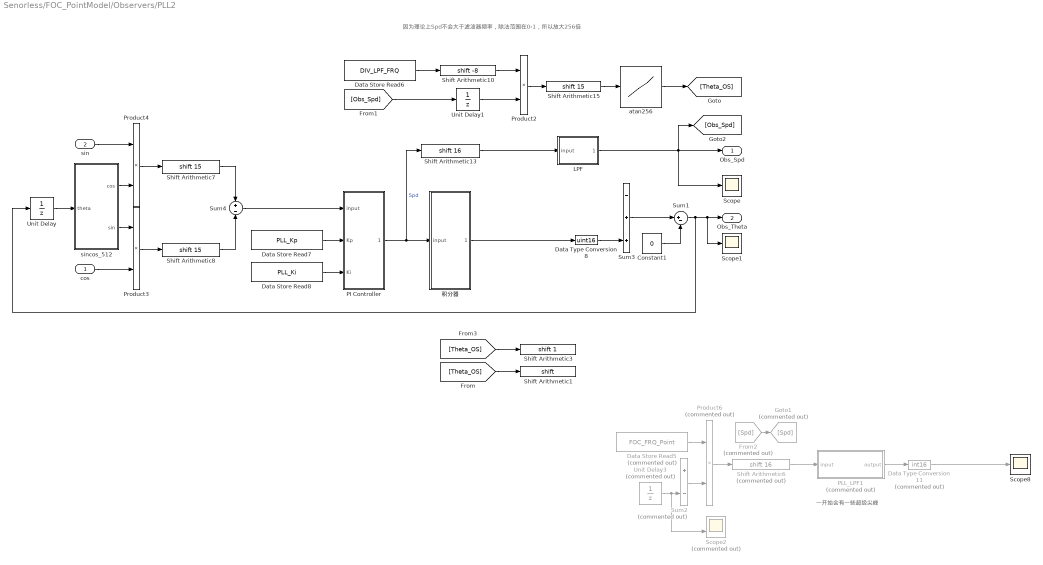
== system Senorless/FOC_PointModel/Observers/PLL2 ==
  note: 因为理论上Spd不会大于滤波器频率，除法范围在0-1，所以放大256倍
  note: 一开始会有一些超级尖峰
  cos : Inport
  sin : Inport  Port=2
  Constant1 : Constant  Value=0  OutDataTypeStr=uint16
  Data Store Read5 : DataStoreRead  Commented=on  DataStoreName=FOC_FRQ_Point  IndexOptions=Index vector (dialog)  Indices=1  OutputSizes=1
  Data Store Read6 : DataStoreRead  DataStoreName=DIV_LPF_FRQ  IndexOptions=Index vector (dialog)  Indices=1  OutputSizes=1
  Data Store Read7 : DataStoreRead  DataStoreName=PLL_Kp  IndexOptions=Index vector (dialog)  Indices=1  OutputSizes=1
  Data Store Read8 : DataStoreRead  DataStoreName=PLL_Ki  IndexOptions=Index vector (dialog)  Indices=1  OutputSizes=1
  Data Type Conversion11 : DataTypeConversion  Commented=on  OutDataTypeStr=int16  SaturateOnIntegerOverflow=off
  Data Type Conversion8 : DataTypeConversion  OutDataTypeStr=uint16  SaturateOnIntegerOverflow=off
  From2 : From  Commented=on  GotoTag=Spd
  Goto1 : Goto  Commented=on  GotoTag=Spd
  LPF : Subsystem  TreatAsAtomicUnit=on
  PI Controller : Subsystem
      settings: MinAlgLoopOccurrences=on
  PLL_LPF1 : Subsystem  Commented=on  TreatAsAtomicUnit=on
  Product2 : Product  OutDataTypeStr=int32  RndMeth=Zero
  Product3 : Product  OutDataTypeStr=int32  RndMeth=Zero
  Product4 : Product  OutDataTypeStr=int32  RndMeth=Zero
  Product6 : Product  Commented=on  OutDataTypeStr=int32  RndMeth=Zero
  Scope : Scope
  Scope1 : Scope
  Scope2 : Scope  Commented=on  NumInputPorts=2
  Scope8 : Scope
  Shift Arithmetic1 : ArithShift
  Shift Arithmetic10 : ArithShift  BitShiftNumber=-8
  Shift Arithmetic13 : ArithShift  BitShiftNumber=16
  Shift Arithmetic15 : ArithShift  BitShiftNumber=15
  Shift Arithmetic3 : ArithShift  BitShiftNumber=1
  Shift Arithmetic6 : ArithShift  Commented=on  BitShiftNumber=16
  Shift Arithmetic7 : ArithShift  BitShiftNumber=15
  Shift Arithmetic8 : ArithShift  BitShiftNumber=15
  Sum1 : Sum  Inputs=|+-  AccumDataTypeStr=uint16  OutDataTypeStr=uint16  RndMeth=Zero
  Sum2 : Sum  Commented=on  Inputs=+-  OutDataTypeStr=int16  RndMeth=Zero
  Sum3 : Sum  Inputs=-++  AccumDataTypeStr=uint16  OutDataTypeStr=uint16  RndMeth=Zero
  Sum4 : Sum  Inputs=+-
  Unit Delay : UnitDelay  SampleTime=-1  HasFrameUpgradeWarning=on
  Unit Delay1 : UnitDelay  SampleTime=-1  HasFrameUpgradeWarning=on
  Unit Delay3 : UnitDelay  Commented=on  SampleTime=-1  HasFrameUpgradeWarning=on
  atan256 : Lookup_n-D  NumberOfTableDimensions=1  BreakpointsSpecification=Even spacing  BreakpointsForDimension1=[-5:5]  UseOneInputPortForAllInputData=on  Table=uint16(16384*atan(linspace(0,1,256)))  TableDataTypeStr=uint16  InterpMethod=Flat  RemoveProtectionInput=on  InternalRulePriority=Speed  OutDataTypeStr=uint16  RndMeth=Zero
  sincos_512 : Subsystem
  积分器 : Subsystem
      settings: MinAlgLoopOccurrences=on
  Obs_Spd : Outport
  Obs_Theta : Outport  Port=2
  wires:
  Sum1/1 -> Unit Delay/1, Scope1/1, Obs_Theta/1
  Shift Arithmetic10/1 -> Product2/1
  Shift Arithmetic15/1 -> atan256/1
  atan256/1 -> [Theta_OS]
  Unit Delay1/1 -> Product2/2
  Data Store Read6/1 -> Shift Arithmetic10/1
  [Obs_Spd] -> Unit Delay1/1
  Product2/1 -> Shift Arithmetic15/1
  Sum4/1 -> PI Controller/1(input)
  sincos_512/2(sin) -> Product3/1
  Product3/1 -> Shift Arithmetic8/1
  Shift Arithmetic8/1 -> Sum4/2
  sincos_512/1(cos) -> Product4/2
  cos/1 -> Product3/2
  sin/1 -> Product4/1
  Product4/1 -> Shift Arithmetic7/1
  Shift Arithmetic7/1 -> Sum4/1
  LPF/1(output) -> Scope/1, Obs_Spd/1, [Obs_Spd]
  Shift Arithmetic13/1 -> LPF/1(input)
  Constant1/1 -> Sum1/2
  [Theta_OS] -> Shift Arithmetic1/1
  [Theta_OS] -> Shift Arithmetic3/1
  Data Type Conversion11/1 -> Scope8/1
  PLL_LPF1/1(output) -> Data Type Conversion11/1
  PI Controller/1(output) -> Shift Arithmetic13/1, 积分器/1(input)  "Spd"
  Data Type Conversion8/1 -> Sum3/3
  Shift Arithmetic6/1 -> PLL_LPF1/1(input)
  积分器/1(output) -> Data Type Conversion8/1
  Data Store Read7/1 -> PI Controller/2(Kp)
  Data Store Read5/1 -> Product6/1
  Product6/1 -> Shift Arithmetic6/1
  Unit Delay3/1 -> Sum2/2, Scope2/2
  Sum2/1 -> Product6/2
  From2/1 -> Goto1/1
  Data Store Read8/1 -> PI Controller/3(Ki)
  Sum3/1 -> Sum1/1
  Unit Delay/1 -> sincos_512/1(theta)
